simulink model "Motion_planner_Street_Drone"  (R2019b)
settings: Solver=FixedStepAuto  StartTime=0.0  StopTime=25  FixedStep=0.0075  MaxStep=1e-1  MinStep=1e-3  RelTol=1e-3  AbsTol=1e-4
InitFcn:
  | SD_init1
values from neighbouring files (symbols this model uses):
  cost = [2.71432892747 3.32441927977 3.79268757264 4.85642115368 6.12135035287 7.09825974303 9.57278659789 1.55754789407 1.51399555616 2.57723707661 3.8468529147 4.8336387623 ... (2430 elements, 1x2430)]    [matlab.mat]
  Front_brake = [0 2.2085352751 4.15209150797 6.12733711785 8.16604105928 9.79119154879 12.1808659635 14.1242630413 16.1155522836 18.1386900579 20.0839213981 22.1313006548 ... (68 elements, 34x2)]    [Front_brake.mat]
  N = size(X,1)    [curvature.m]
  obsx = [dx1 dx2 dx3 dx4]'    [dynamic_collison.m]    (also in dynamic_detection1.m = [x1 x2 x3 x4]')
  obsy = [dy1 dy2 dy3 dy4]'    [dynamic_collison.m]    (also in dynamic_detection1.m = [y1 y2 y3 y4]')
  x = obs_path(i,1)    [dynamic_collison.m]    (also in dynamic_detection1.m)
  X = [X]    [curvature.m]
  y = obs_path(i,2)    [dynamic_collison.m]    (also in dynamic_detection1.m)
undefined symbols (not defined in the file or in its folder): d, dfin, dini, Ki, Kp, L_0f, lookahead_time, lookahead_time_rev, Rear_brake, sigbuilder_block, steer_ratio, steer_sens, tfin, tini, TPS_0, xfin, Y, yfin, Z
libraries: sm_lib x290, nesl_utility x136, simulink x6, vrlib x2, powerlib_meascontrol x2
(part 12 of 14)

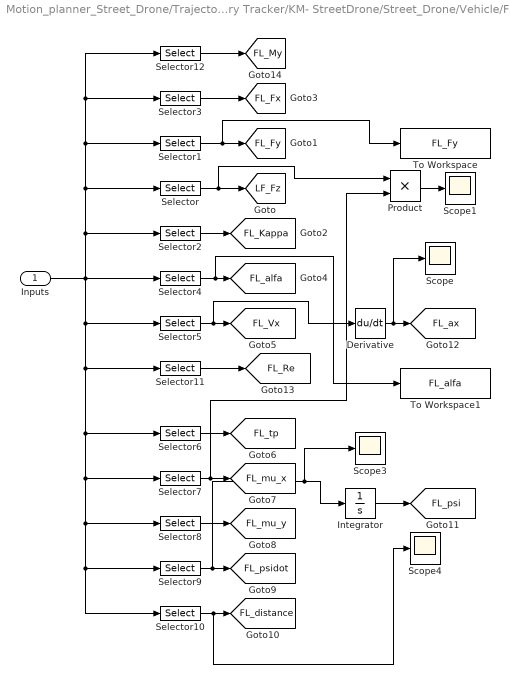
== system Motion_planner_Street_Drone/Trajectory Tracker/KM- StreetDrone/Street_Drone/Vehicle/FL_Wheel/For Validation ==
  Inputs : Inport
  Derivative : Derivative
  Integrator : Integrator
  Product : Product
  Scope{,1,3..4} (4 alike) : Scope
  Selector : Selector  InputPortWidth=40  IndexOptions=Index vector (dialog)  Indices=[3]  OutputSizes=1
  Selector1 : Selector  InputPortWidth=40  IndexOptions=Index vector (dialog)  Indices=[2]  OutputSizes=1
  Selector10 : Selector  InputPortWidth=40  IndexOptions=Index vector (dialog)  Indices=[28]  OutputSizes=1
  Selector11 : Selector  InputPortWidth=40  IndexOptions=Index vector (dialog)  Indices=[13]  OutputSizes=1
  Selector12 : Selector  InputPortWidth=40  IndexOptions=Index vector (dialog)  Indices=[5]  OutputSizes=1
  Selector2 : Selector  InputPortWidth=40  IndexOptions=Index vector (dialog)  Indices=[7]  OutputSizes=1
  Selector3 : Selector  InputPortWidth=40  IndexOptions=Index vector (dialog)  Indices=[1]  OutputSizes=1
  Selector4 : Selector  InputPortWidth=40  IndexOptions=Index vector (dialog)  Indices=[8]  OutputSizes=1
  Selector5 : Selector  InputPortWidth=40  IndexOptions=Index vector (dialog)  Indices=[11]  OutputSizes=1
  Selector6 : Selector  InputPortWidth=40  IndexOptions=Index vector (dialog)  Indices=[16]  OutputSizes=1
  Selector7 : Selector  InputPortWidth=40  IndexOptions=Index vector (dialog)  Indices=[17]  OutputSizes=1
  Selector8 : Selector  InputPortWidth=40  IndexOptions=Index vector (dialog)  Indices=[18]  OutputSizes=1
  Selector9 : Selector  InputPortWidth=40  IndexOptions=Index vector (dialog)  Indices=[24]  OutputSizes=1
  To Workspace : ToWorkspace  VariableName=FL_Fy  SampleTime=-1
  To Workspace1 : ToWorkspace  VariableName=FL_alfa  SampleTime=-1
  tag scope: FL_Fx=global, FL_Fy=global, FL_Kappa=global, FL_My=global, FL_Re=global, FL_Vx=global, FL_alfa=global, FL_ax=global, FL_distance=global, FL_mu_x=global, FL_mu_y=global, FL_psi=global, FL_psidot=global, FL_tp=global, LF_Fz=global
  wires:
  Selector12/1 -> [FL_My]
  Product/1 -> Scope1/1
  Derivative/1 -> [FL_ax], Scope/1
  Integrator/1 -> [FL_psi]
  Selector10/1 -> Scope4/1, [FL_distance]
  Inputs/1 -> Selector4/1, Selector2/1, Selector/1, Selector1/1, Selector3/1, Selector12/1, Selector5/1, Selector6/1, Selector7/1, Selector8/1, Selector9/1, Selector10/1, Selector11/1
  Selector9/1 -> [FL_psidot], Scope3/1, Integrator/1
  Selector8/1 -> [FL_mu_y]
  Selector7/1 -> [FL_mu_x], Product/2
  Selector6/1 -> [FL_tp]
  Selector5/1 -> [FL_Vx], Derivative/1
  Selector4/1 -> To Workspace1/1, [FL_alfa]
  Selector3/1 -> [FL_Fx]
  Selector2/1 -> [FL_Kappa]
  Selector1/1 -> To Workspace/1, [FL_Fy]
  Selector/1 -> [LF_Fz], Product/1
  Selector11/1 -> [FL_Re]

== system Motion_planner_Street_Drone/Trajectory Tracker/KM- StreetDrone/Street_Drone/Vehicle/FL_Wheel/Non-moving road ==
  omega2 : Constant  Value=zeros(18,1)
  road : Outport
  wires:
  omega2/1 -> road/1

== system Motion_planner_Street_Drone/Trajectory Tracker/KM- StreetDrone/Street_Drone/Vehicle/FL_Wheel/Scaling factors ==
  s_LKX : Constant  Value=LKX
  s_LKY : Constant  Value=LKY
  s_LKYC : Constant  Value=LKYC
  s_LKZC : Constant  Value=LKZC
  s_LMUX : Constant  Value=LMUX
  s_LMUY : Constant  Value=LMUY
  s_LTR : Constant  Value=LTR
  scaling_vector : Mux  Inputs=7
  scaling : Outport
  wires:
  s_LMUX/1 -> scaling_vector/1
  s_LKX/1 -> scaling_vector/2
  s_LMUY/1 -> scaling_vector/3
  s_LKY/1 -> scaling_vector/4
  s_LKYC/1 -> scaling_vector/5
  s_LTR/1 -> scaling_vector/6
  s_LKZC/1 -> scaling_vector/7
  scaling_vector/1 -> scaling/1

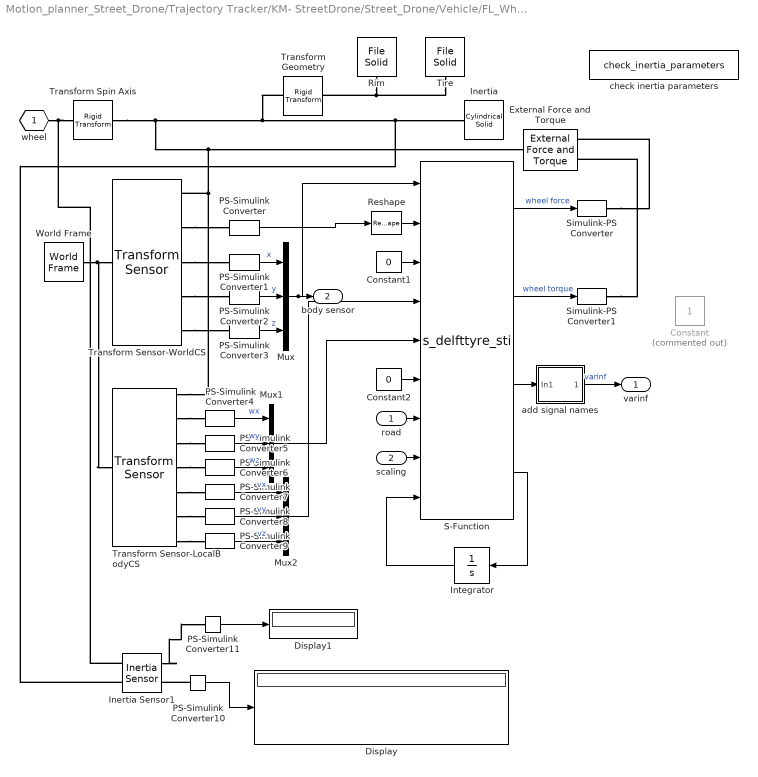
== system Motion_planner_Street_Drone/Trajectory Tracker/KM- StreetDrone/Street_Drone/Vehicle/FL_Wheel/SimMechanics2G Wheel + tyre ==
  road : Inport
  scaling : Inport  Port=2
  Constant : Constant  Commented=on
  Constant1 : Constant  Value=0
  Constant2 : Constant  Value=0
  Display : Display
  Display1 : Display
  External Force and Torque : sm_lib/Forces and Torques/External Force and Torque  ForceResolutionFrame=AttachedFrame  EnableForceX=off  EnableForceY=off  EnableForceZ=off  EnableForce=on  TorqueResolutionFrame=AttachedFrame  EnableTorqueX=off  EnableTorqueY=off  EnableTorqueZ=off  EnableTorque=on
  Inertia : sm_lib/Body Elements/Cylindrical Solid  GraphicAmbientColor=[0.15 0.15 0.15 1.0]  BasedOnType=Density  CenterOfMass=[0 0 0]  CenterOfMassUnits=m  GraphicDiffuseColor=[0.2 0.8 1.0]  CylinderLength=0.001  CylinderLengthUnits=m  CylinderRadius=0.001  CylinderRadiusUnits=m  Density=1000  DensityUnits=kg/(m^3)  DoExposeReferenceFrame=on  GraphicEmissiveColor=[0.0 0.0 0.0 1.0]  ExportEntireGeometry=off  SerializedFrames=<Frames/>  MarkerShape=Sphere  MarkerSize=10  GraphicType=FromGeometry  InertiaType=Custom  Mass=mass  MassUnits=kg  MomentsOfInertia=[Imat(1,1) Imat(2,2) Imat(3,3)]  MomentsOfInertiaUnits=kg*m^2  GraphicOpacity=1.0  ProductsOfInertia=[0 0 0]  ProductsOfInertiaUnits=kg*m^2  GraphicShininess=75  GraphicSpecularColor=[0.5 0.5 0.5 1.0]  GraphicVisPropType=SimpleVisualProperties
  Inertia Sensor1 : sm_lib/Body Elements/Inertia Sensor  SensorExtent=BodyGroup  SpanWeldJoints=off  ExcludeGroundedBodies=off  MeasurementFrame=Custom  SenseMass=on  SenseCenterOfMass=off  SenseInertiaMatrix=on  SenseCenteredInertiaMatrix=off  SensePrincipalInertiaMatrix=off  SenseRotationMatrix=off  GraphicType=PrincipalInertiaFrame  PrincipalInertiaFrameSize=20  GraphicVisPropType=SimpleVisualProperties  GraphicDiffuseColor=[0.5 0.5 0.5]  GraphicSpecularColor=[0.5 0.5 0.5 1.0]  GraphicAmbientColor=[0.15 0.15 0.15 1.0]  GraphicEmissiveColor=[0.0 0.0 0.0 1.0]  GraphicShininess=75  GraphicOpacity=1.0
      settings: SourceProductBaseCode=MS
  Integrator : Integrator  InitialCondition=zeros(1,40)
  Mux : Mux  Inputs=3
  Mux1 : Mux  Inputs=3
  Mux2 : Mux  Inputs=3
  PS-Simulink Converter{,1..9} (10 alike) : nesl_utility/PS-Simulink Converter  PhysicalDomain=network_engine_domain  SubClassName=ps_output  LeftPortType=input  RightPortType=output  PseudoPeriodic=off  Frequencies=[]  Unit=1  AffineConversion=off
  PS-Simulink Converter10 : nesl_utility/PS-Simulink Converter  PhysicalDomain=network_engine_domain  SubClassName=ps_output  LeftPortType=input  RightPortType=output  PseudoPeriodic=off  Frequencies=[]  Unit=inherit  AffineConversion=off
  PS-Simulink Converter11 : nesl_utility/PS-Simulink Converter  PhysicalDomain=network_engine_domain  SubClassName=ps_output  LeftPortType=input  RightPortType=output  PseudoPeriodic=off  Frequencies=[]  Unit=inherit  AffineConversion=off
  Reshape : Reshape
  Rim : sm_lib/Body Elements/File Solid  ExtGeomFileName=D:\Project\PATH PLANNER STREET DRONE - 618341\CAD geometry\Rim_Front.stl  UnitType=Custom  ExtGeomFileUnits=mm  StepReaderType=HEX  ExportEntireGeometry=off  InertiaType=Custom  Mass=0  MassUnits=kg  CenterOfMass=[0 0 0]  CenterOfMassUnits=m  MomentsOfInertia=[0 0 0]  MomentsOfInertiaUnits=kg*m^2  ProductsOfInertia=[0 0 0]  ProductsOfInertiaUnits=kg*m^2  BasedOnType=Density  Density=1000  DensityUnits=kg/(m^3)  DoExposeReferenceFrame=on  SerializedFrames=<Frames/>  GraphicType=FromGeometry  MarkerShape=Sphere  MarkerSize=10  MarkerSizeUnits=m  GraphicVisPropType=SimpleVisualProperties  GraphicDiffuseColor=[0.8 0.8 0.8]  GraphicSpecularColor=[0.5 0.5 0.5 1.0]  GraphicAmbientColor=[0.15 0.15 0.15 1.0]  GraphicEmissiveColor=[0.0 0.0 0.0 1.0]  GraphicShininess=75  GraphicOpacity=1.0
  S-Function : S-Function  FunctionName=s_delfttyre_sti  Parameters=iswtch idtyre idroad tpfname_dummy rdfname typarr  SFunctionDeploymentMode=off  EnableBusSupport=off
  Simulink-PS Converter : nesl_utility/Simulink-PS Converter  PhysicalDomain=network_engine_domain  SubClassName=ps_input  LeftPortType=input  RightPortType=output  PseudoPeriodic=off  Frequencies=[]  NoiseDistribution=none  NoiseParameters=[]  Unit=1  AffineConversion=off  FilteringAndDerivatives=zero  SimscapeFilterOrder=1  InputFilterTimeConstant=0.001  UdotUserProvided=1
  Simulink-PS Converter1 : nesl_utility/Simulink-PS Converter  PhysicalDomain=network_engine_domain  SubClassName=ps_input  LeftPortType=input  RightPortType=output  PseudoPeriodic=off  Frequencies=[]  NoiseDistribution=none  NoiseParameters=[]  Unit=1  AffineConversion=off  FilteringAndDerivatives=zero  SimscapeFilterOrder=1  InputFilterTimeConstant=0.001  UdotUserProvided=1
  Tire : sm_lib/Body Elements/File Solid  ExtGeomFileName=D:\Project\PATH PLANNER STREET DRONE - 618341\CAD geometry\Tire_Front.stl  UnitType=Custom  ExtGeomFileUnits=mm  StepReaderType=HEX  ExportEntireGeometry=off  InertiaType=Custom  Mass=0  MassUnits=kg  CenterOfMass=[0 0 0]  CenterOfMassUnits=m  MomentsOfInertia=[0 0 0]  MomentsOfInertiaUnits=kg*m^2  ProductsOfInertia=[0 0 0]  ProductsOfInertiaUnits=kg*m^2  BasedOnType=Density  Density=1000  DensityUnits=kg/(m^3)  DoExposeReferenceFrame=on  SerializedFrames=<Frames/>  GraphicType=FromGeometry  MarkerShape=Sphere  MarkerSize=10  MarkerSizeUnits=m  GraphicVisPropType=SimpleVisualProperties  GraphicDiffuseColor=[0.5 0.5 0.5]  GraphicSpecularColor=[0.5 0.5 0.5 1.0]  GraphicAmbientColor=[0.15 0.15 0.15 1.0]  GraphicEmissiveColor=[0.0 0.0 0.0 1.0]  GraphicShininess=75  GraphicOpacity=1.0
  Transform Geometry : sm_lib/Frames and Transforms/Rigid Transform  TranslationMethod=StandardAxis  TranslationStandardOffset=(1-2*fliplr)*0.125  TranslationLengthUnit=m  TranslationStandardAxis=+Y  TranslationCartesianOffset=[0 0 0]  TranslationROffset=0  TranslationROffsetUnits=m  TranslationZOffset=0  TranslationZOffsetUnits=m  TranslationThetaOffset=0  TranslationThetaOffsetUnits=deg  RotationMethod=StandardAxis  RotationAngleUnits=deg  RotationStandardAxis=+X  RotationAngle=fliplr*180-90  RotationArbitraryAxis=[0 0 1]  FollAlignAxisA=+X  BaseAlignAxisA=+Y  FollAlignAxisB=+Y  BaseAlignAxisB=+Z  RotationSequenceAxes=FollowerAxes  RotationSequence=XYX  RotationSequenceAngles=[0 0 0]  RotationSequenceAnglesUnits=deg  RotationMatrix=[1 0 0; 0 1 0; 0 0 1]
  Transform Sensor-LocalBodyCS : sm_lib/Frames and Transforms/Transform Sensor  MeasurementFrame=NonRotatingFollower  SenseAngle=off  SenseAxis=off  SenseAngle1=off  SenseAngle2=off  SenseAngle3=off  SenseQ=off  SenseR=off  SenseOmegaX=on  SenseOmegaY=on  SenseOmegaZ=on  SenseOmega1=off  SenseOmega2=off  SenseOmega3=off  SenseQDot=off  SenseRDot=off  SenseAlphaX=off  SenseAlphaY=off  SenseAlphaZ=off  SenseAlpha1=off  SenseAlpha2=off  SenseAlpha3=off  SenseQDDot=off  SenseRDDot=off  SenseX=off  SenseY=off  SenseZ=off  SenseRad=off  SenseAzim=off  SenseDist=off  SenseInc=off  SenseXDot=on  SenseYDot=on  SenseZDot=on  SenseRadDot=off  SenseAzimDot=off  SenseDistDot=off  SenseIncDot=off  SenseXDDot=off  SenseYDDot=off  SenseZDDot=off  SenseRadDDot=off  SenseAzimDDot=off  SenseDistDDot=off  SenseIncDDot=off
  Transform Sensor-WorldCS : sm_lib/Frames and Transforms/Transform Sensor  MeasurementFrame=World  SenseAngle=off  SenseAxis=off  SenseAngle1=off  SenseAngle2=off  SenseAngle3=off  SenseQ=off  SenseR=on  SenseOmegaX=off  SenseOmegaY=off  SenseOmegaZ=off  SenseOmega1=off  SenseOmega2=off  SenseOmega3=off  SenseQDot=off  SenseRDot=off  SenseAlphaX=off  SenseAlphaY=off  SenseAlphaZ=off  SenseAlpha1=off  SenseAlpha2=off  SenseAlpha3=off  SenseQDDot=off  SenseRDDot=off  SenseX=on  SenseY=on  SenseZ=on  SenseRad=off  SenseAzim=off  SenseDist=off  SenseInc=off  SenseXDot=off  SenseYDot=off  SenseZDot=off  SenseRadDot=off  SenseAzimDot=off  SenseDistDot=off  SenseIncDot=off  SenseXDDot=off  SenseYDDot=off  SenseZDDot=off  SenseRadDDot=off  SenseAzimDDot=off  SenseDistDDot=off  SenseIncDDot=off
  Transform Spin Axis : sm_lib/Frames and Transforms/Rigid Transform  TranslationMethod=None  TranslationStandardOffset=0  TranslationLengthUnit=m  TranslationStandardAxis=+Z  TranslationCartesianOffset=[0 0 0]  TranslationROffset=0  TranslationROffsetUnits=m  TranslationZOffset=0  TranslationZOffsetUnits=m  TranslationThetaOffset=0  TranslationThetaOffsetUnits=deg  RotationMethod=StandardAxis  RotationAngleUnits=deg  RotationStandardAxis=-X  RotationAngle=90  RotationArbitraryAxis=[0 0 1]  FollAlignAxisA=+X  BaseAlignAxisA=+Y  FollAlignAxisB=+Y  BaseAlignAxisB=+Z  RotationSequenceAxes=FollowerAxes  RotationSequence=XYX  RotationSequenceAngles=[0 0 0]  RotationSequenceAnglesUnits=deg  RotationMatrix=[1 0 0; 0 1 0; 0 0 1]
  World Frame : sm_lib/Frames and Transforms/World Frame
  add signal names : Subsystem
  check inertia parameters : M-S-Function  Priority=1  FunctionName=check_inertia_parameters  Parameters=tpfname1, rdfname1, typarr1  mask{tpfname1=tpfname_dummy, rdfname1=rdfname, typarr1=typarr}
      mask prompts: tpfname1 "Tyre Property File"; rdfname1 "Road Data File"; typarr1 "typarr"
      mask help: Checks Inertia parameters as calculated in mask
  wheel : PMIOPort  Side=Left
  varinf : Outport
  body sensor : Outport  Port=2
  wires:
  PS-Simulink Converter11/1 -> Display1/1
  PS-Simulink Converter10/1 -> Display/1
  Constant2/1 -> S-Function/6
  Mux2/1 -> S-Function/4
  Mux1/1 -> S-Function/5
  PS-Simulink Converter/1 -> Reshape/1
  S-Function/4 -> Integrator/1
  S-Function/3 -> add signal names/1(In1)
  add signal names/1(Out1) -> varinf/1  "varinf"
  road/1 -> S-Function/7
  scaling/1 -> S-Function/8
  Integrator/1 -> S-Function/9
  Constant1/1 -> S-Function/3
  PS-Simulink Converter1/1 -> Mux/1  "x"
  PS-Simulink Converter2/1 -> Mux/2  "y"
  PS-Simulink Converter3/1 -> Mux/3  "z"
  PS-Simulink Converter4/1 -> Mux1/1  "wx"
  PS-Simulink Converter5/1 -> Mux1/2  "wy"
  PS-Simulink Converter6/1 -> Mux1/3  "wz"
  PS-Simulink Converter7/1 -> Mux2/1  "vx"
  PS-Simulink Converter8/1 -> Mux2/2  "vy"
  PS-Simulink Converter9/1 -> Mux2/3  "vz"
  Mux/1 -> body sensor/1, S-Function/1
  S-Function/2 -> Simulink-PS Converter1/1  "wheel torque"
  S-Function/1 -> Simulink-PS Converter/1  "wheel force"
  Reshape/1 -> S-Function/2
  connections:
  Inertia Sensor1/RConn1 -- PS-Simulink Converter11/LConn1
  PS-Simulink Converter10/LConn1 -- Inertia Sensor1/RConn2
  Inertia Sensor1/LConn1 -- wheel/RConn1 -- Transform Spin Axis/RConn1
  Simulink-PS Converter1/RConn1 -- External Force and Torque/LConn2
  Simulink-PS Converter/RConn1 -- External Force and Torque/LConn1
  Transform Sensor-WorldCS/RConn2 -- PS-Simulink Converter/LConn1
  Transform Sensor-WorldCS/RConn3 -- PS-Simulink Converter1/LConn1
  Transform Sensor-WorldCS/RConn4 -- PS-Simulink Converter2/LConn1
  Transform Sensor-WorldCS/RConn5 -- PS-Simulink Converter3/LConn1
  Transform Sensor-LocalBodyCS/RConn2 -- PS-Simulink Converter4/LConn1
  Transform Sensor-LocalBodyCS/RConn3 -- PS-Simulink Converter5/LConn1
  Transform Sensor-LocalBodyCS/RConn4 -- PS-Simulink Converter6/LConn1
  Transform Sensor-LocalBodyCS/RConn5 -- PS-Simulink Converter7/LConn1
  Transform Sensor-LocalBodyCS/RConn6 -- PS-Simulink Converter8/LConn1
  Transform Sensor-LocalBodyCS/RConn7 -- PS-Simulink Converter9/LConn1
  Tire/RConn1 -- Rim/RConn1 -- Transform Geometry/RConn1
  Inertia Sensor1/LConn2 -- Transform Geometry/LConn1 -- External Force and Torque/RConn1 -- Transform Sensor-LocalBodyCS/RConn1 -- Transform Sensor-WorldCS/RConn1 -- Transform Spin Axis/LConn1 -- Inertia/RConn1
  Transform Sensor-LocalBodyCS/LConn1 -- World Frame/RConn1 -- Transform Sensor-WorldCS/LConn1

== system Motion_planner_Street_Drone/Trajectory Tracker/KM- StreetDrone/Street_Drone/Vehicle/FR_Suspension/steering_angle_measurement ==
  Integrator1 : Integrator
  PS-Simulink Converter3 : nesl_utility/PS-Simulink Converter  PhysicalDomain=network_engine_domain  SubClassName=ps_output  LeftPortType=input  RightPortType=output  PseudoPeriodic=off  Frequencies=[]  Unit=inherit  AffineConversion=off
  PS-Simulink Converter4 : nesl_utility/PS-Simulink Converter  PhysicalDomain=network_engine_domain  SubClassName=ps_output  LeftPortType=input  RightPortType=output  PseudoPeriodic=off  Frequencies=[]  Unit=inherit  AffineConversion=off
  Scope2 : Scope  NumInputPorts=2
  Transform Sensor2 : sm_lib/Frames and Transforms/Transform Sensor  MeasurementFrame=Base  SenseAngle=off  SenseAxis=off  SenseAngle1=off  SenseAngle2=off  SenseAngle3=off  SenseQ=off  SenseR=off  SenseOmegaX=off  SenseOmegaY=on  SenseOmegaZ=on  SenseOmega1=off  SenseOmega2=off  SenseOmega3=off  SenseQDot=off  SenseRDot=off  SenseAlphaX=off  SenseAlphaY=off  SenseAlphaZ=off  SenseAlpha1=off  SenseAlpha2=off  SenseAlpha3=off  SenseQDDot=off  SenseRDDot=off  SenseX=off  SenseY=off  SenseZ=off  SenseRad=off  SenseAzim=off  SenseDist=off  SenseInc=off  SenseXDot=off  SenseYDot=off  SenseZDot=off  SenseRadDot=off  SenseAzimDot=off  SenseDistDot=off  SenseIncDot=off  SenseXDDot=off  SenseYDDot=off  SenseZDDot=off  SenseRadDDot=off  SenseAzimDDot=off  SenseDistDDot=off  SenseIncDDot=off
  vehicle : PMIOPort  Side=Left
  suspension_z-axis : PMIOPort  Port=2  Side=Right
  tag scope: Del_R=global
  wires:
  PS-Simulink Converter3/1 -> Integrator1/1
  PS-Simulink Converter4/1 -> Scope2/1
  Integrator1/1 -> Scope2/2, [Del_R]
  connections:
  PS-Simulink Converter4/LConn1 -- Transform Sensor2/RConn2
  suspension_z-axis/RConn1 -- Transform Sensor2/RConn1
  Transform Sensor2/LConn1 -- vehicle/RConn1
  PS-Simulink Converter3/LConn1 -- Transform Sensor2/RConn3

== system Motion_planner_Street_Drone/Trajectory Tracker/KM- StreetDrone/Street_Drone/Vehicle/FR_Wheel/For Validation ==
  Inputs : Inport
  Derivative : Derivative
  Integrator : Integrator
  Scope : Scope
  Selector : Selector  InputPortWidth=40  IndexOptions=Index vector (dialog)  Indices=[3]  OutputSizes=1
  Selector1 : Selector  InputPortWidth=40  IndexOptions=Index vector (dialog)  Indices=[2]  OutputSizes=1
  Selector10 : Selector  InputPortWidth=40  IndexOptions=Index vector (dialog)  Indices=[28]  OutputSizes=1
  Selector11 : Selector  InputPortWidth=40  IndexOptions=Index vector (dialog)  Indices=[13]  OutputSizes=1
  Selector12 : Selector  InputPortWidth=40  IndexOptions=Index vector (dialog)  Indices=[5]  OutputSizes=1
  Selector2 : Selector  InputPortWidth=40  IndexOptions=Index vector (dialog)  Indices=[7]  OutputSizes=1
  Selector3 : Selector  InputPortWidth=40  IndexOptions=Index vector (dialog)  Indices=[1]  OutputSizes=1
  Selector4 : Selector  InputPortWidth=40  IndexOptions=Index vector (dialog)  Indices=[8]  OutputSizes=1
  Selector5 : Selector  InputPortWidth=40  IndexOptions=Index vector (dialog)  Indices=[11]  OutputSizes=1
  Selector6 : Selector  InputPortWidth=40  IndexOptions=Index vector (dialog)  Indices=[16]  OutputSizes=1
  Selector7 : Selector  InputPortWidth=40  IndexOptions=Index vector (dialog)  Indices=[17]  OutputSizes=1
  Selector8 : Selector  InputPortWidth=40  IndexOptions=Index vector (dialog)  Indices=[18]  OutputSizes=1
  Selector9 : Selector  InputPortWidth=40  IndexOptions=Index vector (dialog)  Indices=[24]  OutputSizes=1
  tag scope: FR_Fx=global, FR_Fy=global, FR_Kappa=global, FR_My=global, FR_Re=global, FR_Vx=global, FR_alfa=global, FR_ax=global, FR_distance=global, FR_mu_x=global, FR_mu_y=global, FR_psi=global, FR_psidot=global, FR_tp=global, RF_Fz=global
  wires:
  Selector12/1 -> [FR_My]
  Derivative/1 -> [FR_ax]
  Integrator/1 -> [FR_psi]
  Selector10/1 -> [FR_distance]
  Inputs/1 -> Selector4/1, Selector2/1, Selector/1, Selector1/1, Selector3/1, Selector12/1, Selector5/1, Selector11/1, Selector6/1, Selector7/1, Selector8/1, Selector9/1, Selector10/1
  Selector9/1 -> [FR_psidot], Scope/1, Integrator/1
  Selector8/1 -> [FR_mu_y]
  Selector7/1 -> [FR_mu_x]
  Selector6/1 -> [FR_tp]
  Selector5/1 -> [FR_Vx], Derivative/1
  Selector4/1 -> [FR_alfa]
  Selector3/1 -> [FR_Fx]
  Selector2/1 -> [FR_Kappa]
  Selector1/1 -> [FR_Fy]
  Selector/1 -> [RF_Fz]
  Selector11/1 -> [FR_Re]

== system Motion_planner_Street_Drone/Trajectory Tracker/KM- StreetDrone/Street_Drone/Vehicle/FR_Wheel/Non-moving road ==
  omega2 : Constant  Value=zeros(18,1)
  road : Outport
  wires:
  omega2/1 -> road/1

== system Motion_planner_Street_Drone/Trajectory Tracker/KM- StreetDrone/Street_Drone/Vehicle/FR_Wheel/Scaling factors ==
  s_LKX : Constant  Value=LKX
  s_LKY : Constant  Value=LKY
  s_LKYC : Constant  Value=LKYC
  s_LKZC : Constant  Value=LKZC
  s_LMUX : Constant  Value=LMUX
  s_LMUY : Constant  Value=LMUY
  s_LTR : Constant  Value=LTR
  scaling_vector : Mux  Inputs=7
  scaling : Outport
  wires:
  scaling_vector/1 -> scaling/1
  s_LKZC/1 -> scaling_vector/7
  s_LTR/1 -> scaling_vector/6
  s_LKYC/1 -> scaling_vector/5
  s_LKY/1 -> scaling_vector/4
  s_LMUY/1 -> scaling_vector/3
  s_LKX/1 -> scaling_vector/2
  s_LMUX/1 -> scaling_vector/1

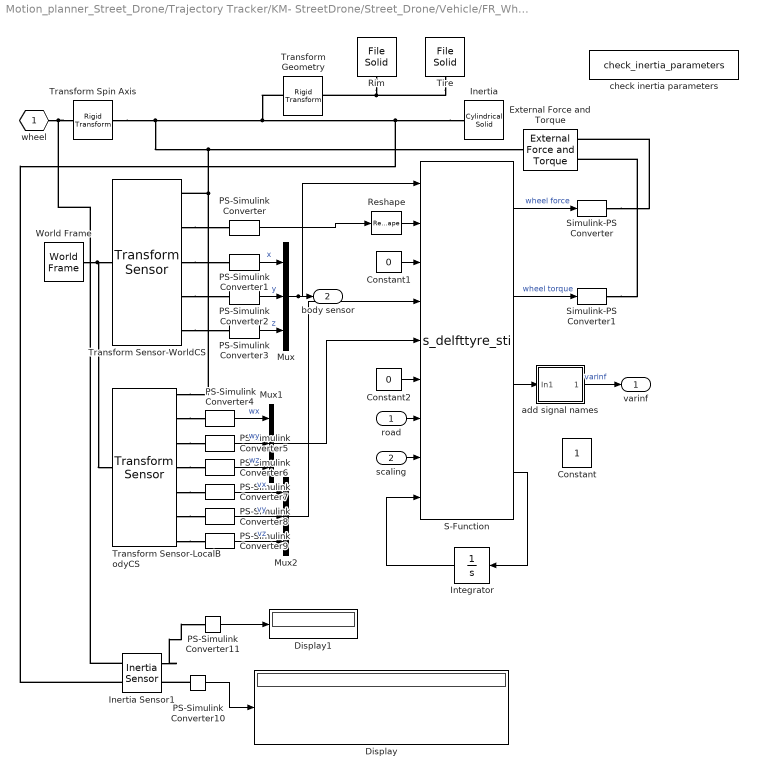
== system Motion_planner_Street_Drone/Trajectory Tracker/KM- StreetDrone/Street_Drone/Vehicle/FR_Wheel/SimMechanics2G Wheel + tyre ==
  road : Inport
  scaling : Inport  Port=2
  Constant : Constant
  Constant1 : Constant  Value=0
  Constant2 : Constant  Value=0
  Display : Display
  Display1 : Display
  External Force and Torque : sm_lib/Forces and Torques/External Force and Torque  ForceResolutionFrame=AttachedFrame  EnableForceX=off  EnableForceY=off  EnableForceZ=off  EnableForce=on  TorqueResolutionFrame=AttachedFrame  EnableTorqueX=off  EnableTorqueY=off  EnableTorqueZ=off  EnableTorque=on
  Inertia : sm_lib/Body Elements/Cylindrical Solid  GraphicAmbientColor=[0.15 0.15 0.15 1.0]  BasedOnType=Density  CenterOfMass=[0 0 0]  CenterOfMassUnits=m  GraphicDiffuseColor=[0.2 0.8 1.0]  CylinderLength=0.001  CylinderLengthUnits=m  CylinderRadius=0.001  CylinderRadiusUnits=m  Density=1000  DensityUnits=kg/(m^3)  DoExposeReferenceFrame=on  GraphicEmissiveColor=[0.0 0.0 0.0 1.0]  ExportEntireGeometry=off  SerializedFrames=<Frames/>  MarkerShape=Sphere  MarkerSize=10  GraphicType=FromGeometry  InertiaType=Custom  Mass=mass  MassUnits=kg  MomentsOfInertia=[Imat(1,1) Imat(2,2) Imat(3,3)]  MomentsOfInertiaUnits=kg*m^2  GraphicOpacity=1.0  ProductsOfInertia=[0 0 0]  ProductsOfInertiaUnits=kg*m^2  GraphicShininess=75  GraphicSpecularColor=[0.5 0.5 0.5 1.0]  GraphicVisPropType=SimpleVisualProperties
  Inertia Sensor1 : sm_lib/Body Elements/Inertia Sensor  SensorExtent=BodyGroup  SpanWeldJoints=off  ExcludeGroundedBodies=off  MeasurementFrame=Custom  SenseMass=on  SenseCenterOfMass=off  SenseInertiaMatrix=on  SenseCenteredInertiaMatrix=off  SensePrincipalInertiaMatrix=off  SenseRotationMatrix=off  GraphicType=PrincipalInertiaFrame  PrincipalInertiaFrameSize=20  GraphicVisPropType=SimpleVisualProperties  GraphicDiffuseColor=[0.5 0.5 0.5]  GraphicSpecularColor=[0.5 0.5 0.5 1.0]  GraphicAmbientColor=[0.15 0.15 0.15 1.0]  GraphicEmissiveColor=[0.0 0.0 0.0 1.0]  GraphicShininess=75  GraphicOpacity=1.0
      settings: SourceProductBaseCode=MS
  Integrator : Integrator  InitialCondition=zeros(1,40)
  Mux : Mux  Inputs=3
  Mux1 : Mux  Inputs=3
  Mux2 : Mux  Inputs=3
  PS-Simulink Converter{,1..9} (10 alike) : nesl_utility/PS-Simulink Converter  PhysicalDomain=network_engine_domain  SubClassName=ps_output  LeftPortType=input  RightPortType=output  PseudoPeriodic=off  Frequencies=[]  Unit=1  AffineConversion=off
  PS-Simulink Converter10 : nesl_utility/PS-Simulink Converter  PhysicalDomain=network_engine_domain  SubClassName=ps_output  LeftPortType=input  RightPortType=output  PseudoPeriodic=off  Frequencies=[]  Unit=inherit  AffineConversion=off
  PS-Simulink Converter11 : nesl_utility/PS-Simulink Converter  PhysicalDomain=network_engine_domain  SubClassName=ps_output  LeftPortType=input  RightPortType=output  PseudoPeriodic=off  Frequencies=[]  Unit=inherit  AffineConversion=off
  Reshape : Reshape
  Rim : sm_lib/Body Elements/File Solid  ExtGeomFileName=D:\Project\PATH PLANNER STREET DRONE - 618341\CAD geometry\Rim_Front.stl  UnitType=Custom  ExtGeomFileUnits=mm  StepReaderType=HEX  ExportEntireGeometry=off  InertiaType=Custom  Mass=0  MassUnits=kg  CenterOfMass=[0 0 0]  CenterOfMassUnits=m  MomentsOfInertia=[0 0 0]  MomentsOfInertiaUnits=kg*m^2  ProductsOfInertia=[0 0 0]  ProductsOfInertiaUnits=kg*m^2  BasedOnType=Density  Density=1000  DensityUnits=kg/(m^3)  DoExposeReferenceFrame=on  SerializedFrames=<Frames/>  GraphicType=FromGeometry  MarkerShape=Sphere  MarkerSize=10  MarkerSizeUnits=m  GraphicVisPropType=SimpleVisualProperties  GraphicDiffuseColor=[0.8 0.8 0.8]  GraphicSpecularColor=[0.5 0.5 0.5 1.0]  GraphicAmbientColor=[0.15 0.15 0.15 1.0]  GraphicEmissiveColor=[0.0 0.0 0.0 1.0]  GraphicShininess=75  GraphicOpacity=1.0
  S-Function : S-Function  FunctionName=s_delfttyre_sti  Parameters=iswtch idtyre idroad tpfname_dummy rdfname typarr  SFunctionDeploymentMode=off  EnableBusSupport=off
  Simulink-PS Converter : nesl_utility/Simulink-PS Converter  PhysicalDomain=network_engine_domain  SubClassName=ps_input  LeftPortType=input  RightPortType=output  PseudoPeriodic=off  Frequencies=[]  NoiseDistribution=none  NoiseParameters=[]  Unit=1  AffineConversion=off  FilteringAndDerivatives=zero  SimscapeFilterOrder=1  InputFilterTimeConstant=0.001  UdotUserProvided=1
  Simulink-PS Converter1 : nesl_utility/Simulink-PS Converter  PhysicalDomain=network_engine_domain  SubClassName=ps_input  LeftPortType=input  RightPortType=output  PseudoPeriodic=off  Frequencies=[]  NoiseDistribution=none  NoiseParameters=[]  Unit=1  AffineConversion=off  FilteringAndDerivatives=zero  SimscapeFilterOrder=1  InputFilterTimeConstant=0.001  UdotUserProvided=1
  Tire : sm_lib/Body Elements/File Solid  ExtGeomFileName=D:\Project\PATH PLANNER STREET DRONE - 618341\CAD geometry\Tire_Front.stl  UnitType=Custom  ExtGeomFileUnits=mm  StepReaderType=HEX  ExportEntireGeometry=off  InertiaType=Custom  Mass=0  MassUnits=kg  CenterOfMass=[0 0 0]  CenterOfMassUnits=m  MomentsOfInertia=[0 0 0]  MomentsOfInertiaUnits=kg*m^2  ProductsOfInertia=[0 0 0]  ProductsOfInertiaUnits=kg*m^2  BasedOnType=Density  Density=1000  DensityUnits=kg/(m^3)  DoExposeReferenceFrame=on  SerializedFrames=<Frames/>  GraphicType=FromGeometry  MarkerShape=Sphere  MarkerSize=10  MarkerSizeUnits=m  GraphicVisPropType=SimpleVisualProperties  GraphicDiffuseColor=[0.5 0.5 0.5]  GraphicSpecularColor=[0.5 0.5 0.5 1.0]  GraphicAmbientColor=[0.15 0.15 0.15 1.0]  GraphicEmissiveColor=[0.0 0.0 0.0 1.0]  GraphicShininess=75  GraphicOpacity=1.0
  Transform Geometry : sm_lib/Frames and Transforms/Rigid Transform  TranslationMethod=StandardAxis  TranslationStandardOffset=(1-2*fliplr)*0.125  TranslationLengthUnit=m  TranslationStandardAxis=+Y  TranslationCartesianOffset=[0 0 0]  TranslationROffset=0  TranslationROffsetUnits=m  TranslationZOffset=0  TranslationZOffsetUnits=m  TranslationThetaOffset=0  TranslationThetaOffsetUnits=deg  RotationMethod=StandardAxis  RotationAngleUnits=deg  RotationStandardAxis=+X  RotationAngle=fliplr*180-90  RotationArbitraryAxis=[0 0 1]  FollAlignAxisA=+X  BaseAlignAxisA=+Y  FollAlignAxisB=+Y  BaseAlignAxisB=+Z  RotationSequenceAxes=FollowerAxes  RotationSequence=XYX  RotationSequenceAngles=[0 0 0]  RotationSequenceAnglesUnits=deg  RotationMatrix=[1 0 0; 0 1 0; 0 0 1]
  Transform Sensor-LocalBodyCS : sm_lib/Frames and Transforms/Transform Sensor  MeasurementFrame=NonRotatingFollower  SenseAngle=off  SenseAxis=off  SenseAngle1=off  SenseAngle2=off  SenseAngle3=off  SenseQ=off  SenseR=off  SenseOmegaX=on  SenseOmegaY=on  SenseOmegaZ=on  SenseOmega1=off  SenseOmega2=off  SenseOmega3=off  SenseQDot=off  SenseRDot=off  SenseAlphaX=off  SenseAlphaY=off  SenseAlphaZ=off  SenseAlpha1=off  SenseAlpha2=off  SenseAlpha3=off  SenseQDDot=off  SenseRDDot=off  SenseX=off  SenseY=off  SenseZ=off  SenseRad=off  SenseAzim=off  SenseDist=off  SenseInc=off  SenseXDot=on  SenseYDot=on  SenseZDot=on  SenseRadDot=off  SenseAzimDot=off  SenseDistDot=off  SenseIncDot=off  SenseXDDot=off  SenseYDDot=off  SenseZDDot=off  SenseRadDDot=off  SenseAzimDDot=off  SenseDistDDot=off  SenseIncDDot=off
  Transform Sensor-WorldCS : sm_lib/Frames and Transforms/Transform Sensor  MeasurementFrame=World  SenseAngle=off  SenseAxis=off  SenseAngle1=off  SenseAngle2=off  SenseAngle3=off  SenseQ=off  SenseR=on  SenseOmegaX=off  SenseOmegaY=off  SenseOmegaZ=off  SenseOmega1=off  SenseOmega2=off  SenseOmega3=off  SenseQDot=off  SenseRDot=off  SenseAlphaX=off  SenseAlphaY=off  SenseAlphaZ=off  SenseAlpha1=off  SenseAlpha2=off  SenseAlpha3=off  SenseQDDot=off  SenseRDDot=off  SenseX=on  SenseY=on  SenseZ=on  SenseRad=off  SenseAzim=off  SenseDist=off  SenseInc=off  SenseXDot=off  SenseYDot=off  SenseZDot=off  SenseRadDot=off  SenseAzimDot=off  SenseDistDot=off  SenseIncDot=off  SenseXDDot=off  SenseYDDot=off  SenseZDDot=off  SenseRadDDot=off  SenseAzimDDot=off  SenseDistDDot=off  SenseIncDDot=off
  Transform Spin Axis : sm_lib/Frames and Transforms/Rigid Transform  TranslationMethod=None  TranslationStandardOffset=0  TranslationLengthUnit=m  TranslationStandardAxis=+Z  TranslationCartesianOffset=[0 0 0]  TranslationROffset=0  TranslationROffsetUnits=m  TranslationZOffset=0  TranslationZOffsetUnits=m  TranslationThetaOffset=0  TranslationThetaOffsetUnits=deg  RotationMethod=StandardAxis  RotationAngleUnits=deg  RotationStandardAxis=-X  RotationAngle=90  RotationArbitraryAxis=[0 0 1]  FollAlignAxisA=+X  BaseAlignAxisA=+Y  FollAlignAxisB=+Y  BaseAlignAxisB=+Z  RotationSequenceAxes=FollowerAxes  RotationSequence=XYX  RotationSequenceAngles=[0 0 0]  RotationSequenceAnglesUnits=deg  RotationMatrix=[1 0 0; 0 1 0; 0 0 1]
  World Frame : sm_lib/Frames and Transforms/World Frame
  add signal names : Subsystem
  check inertia parameters : M-S-Function  Priority=1  FunctionName=check_inertia_parameters  Parameters=tpfname1, rdfname1, typarr1  mask{tpfname1=tpfname_dummy, rdfname1=rdfname, typarr1=typarr}
      mask prompts: tpfname1 "Tyre Property File"; rdfname1 "Road Data File"; typarr1 "typarr"
      mask help: Checks Inertia parameters as calculated in mask
  wheel : PMIOPort  Side=Left
  varinf : Outport
  body sensor : Outport  Port=2
  wires:
  Reshape/1 -> S-Function/2
  S-Function/1 -> Simulink-PS Converter/1  "wheel force"
  S-Function/2 -> Simulink-PS Converter1/1  "wheel torque"
  Mux/1 -> S-Function/1, body sensor/1
  PS-Simulink Converter9/1 -> Mux2/3  "vz"
  PS-Simulink Converter8/1 -> Mux2/2  "vy"
  PS-Simulink Converter7/1 -> Mux2/1  "vx"
  PS-Simulink Converter6/1 -> Mux1/3  "wz"
  PS-Simulink Converter5/1 -> Mux1/2  "wy"
  PS-Simulink Converter4/1 -> Mux1/1  "wx"
  PS-Simulink Converter3/1 -> Mux/3  "z"
  PS-Simulink Converter2/1 -> Mux/2  "y"
  PS-Simulink Converter1/1 -> Mux/1  "x"
  Constant1/1 -> S-Function/3
  Integrator/1 -> S-Function/9
  scaling/1 -> S-Function/8
  road/1 -> S-Function/7
  add signal names/1(Out1) -> varinf/1  "varinf"
  S-Function/3 -> add signal names/1(In1)
  S-Function/4 -> Integrator/1
  PS-Simulink Converter/1 -> Reshape/1
  Mux1/1 -> S-Function/5
  Mux2/1 -> S-Function/4
  Constant2/1 -> S-Function/6
  PS-Simulink Converter10/1 -> Display/1
  PS-Simulink Converter11/1 -> Display1/1
  connections:
  Transform Sensor-WorldCS/LConn1 -- World Frame/RConn1 -- Transform Sensor-LocalBodyCS/LConn1
  Inertia/RConn1 -- Transform Spin Axis/LConn1 -- Transform Sensor-WorldCS/RConn1 -- Transform Sensor-LocalBodyCS/RConn1 -- External Force and Torque/RConn1 -- Transform Geometry/LConn1 -- Inertia Sensor1/LConn2
  Transform Geometry/RConn1 -- Rim/RConn1 -- Tire/RConn1
  Transform Sensor-LocalBodyCS/RConn7 -- PS-Simulink Converter9/LConn1
  Transform Sensor-LocalBodyCS/RConn6 -- PS-Simulink Converter8/LConn1
  Transform Sensor-LocalBodyCS/RConn5 -- PS-Simulink Converter7/LConn1
  Transform Sensor-LocalBodyCS/RConn4 -- PS-Simulink Converter6/LConn1
  Transform Sensor-LocalBodyCS/RConn3 -- PS-Simulink Converter5/LConn1
  Transform Sensor-LocalBodyCS/RConn2 -- PS-Simulink Converter4/LConn1
  Transform Sensor-WorldCS/RConn5 -- PS-Simulink Converter3/LConn1
  Transform Sensor-WorldCS/RConn4 -- PS-Simulink Converter2/LConn1
  Transform Sensor-WorldCS/RConn3 -- PS-Simulink Converter1/LConn1
  Transform Sensor-WorldCS/RConn2 -- PS-Simulink Converter/LConn1
  Simulink-PS Converter/RConn1 -- External Force and Torque/LConn1
  Simulink-PS Converter1/RConn1 -- External Force and Torque/LConn2
  Transform Spin Axis/RConn1 -- wheel/RConn1 -- Inertia Sensor1/LConn1
  PS-Simulink Converter10/LConn1 -- Inertia Sensor1/RConn2
  Inertia Sensor1/RConn1 -- PS-Simulink Converter11/LConn1

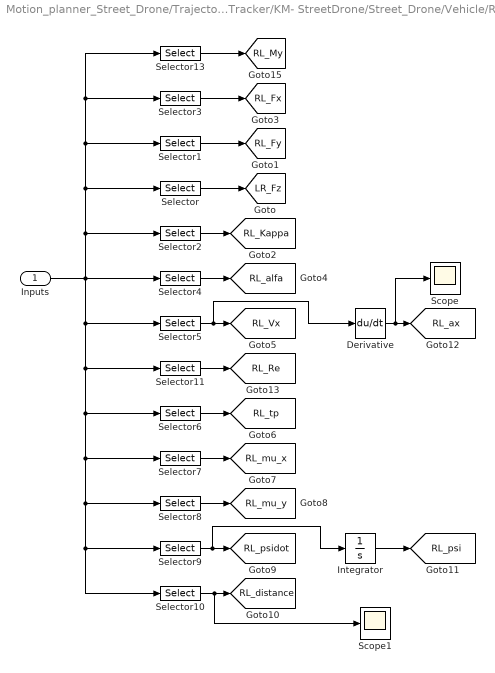
== system Motion_planner_Street_Drone/Trajectory Tracker/KM- StreetDrone/Street_Drone/Vehicle/RL_Wheel/For Validation ==
  Inputs : Inport
  Derivative : Derivative
  Integrator : Integrator
  Scope : Scope
  Scope1 : Scope
  Selector : Selector  InputPortWidth=40  IndexOptions=Index vector (dialog)  Indices=[3]  OutputSizes=1
  Selector1 : Selector  InputPortWidth=40  IndexOptions=Index vector (dialog)  Indices=[2]  OutputSizes=1
  Selector10 : Selector  InputPortWidth=40  IndexOptions=Index vector (dialog)  Indices=[28]  OutputSizes=1
  Selector11 : Selector  InputPortWidth=40  IndexOptions=Index vector (dialog)  Indices=[13]  OutputSizes=1
  Selector13 : Selector  InputPortWidth=40  IndexOptions=Index vector (dialog)  Indices=[5]  OutputSizes=1
  Selector2 : Selector  InputPortWidth=40  IndexOptions=Index vector (dialog)  Indices=[7]  OutputSizes=1
  Selector3 : Selector  InputPortWidth=40  IndexOptions=Index vector (dialog)  Indices=[1]  OutputSizes=1
  Selector4 : Selector  InputPortWidth=40  IndexOptions=Index vector (dialog)  Indices=[8]  OutputSizes=1
  Selector5 : Selector  InputPortWidth=40  IndexOptions=Index vector (dialog)  Indices=[11]  OutputSizes=1
  Selector6 : Selector  InputPortWidth=40  IndexOptions=Index vector (dialog)  Indices=[16]  OutputSizes=1
  Selector7 : Selector  InputPortWidth=40  IndexOptions=Index vector (dialog)  Indices=[17]  OutputSizes=1
  Selector8 : Selector  InputPortWidth=40  IndexOptions=Index vector (dialog)  Indices=[18]  OutputSizes=1
  Selector9 : Selector  InputPortWidth=40  IndexOptions=Index vector (dialog)  Indices=[24]  OutputSizes=1
  tag scope: LR_Fz=global, RL_Fx=global, RL_Fy=global, RL_Kappa=global, RL_My=global, RL_Re=global, RL_Vx=global, RL_alfa=global, RL_ax=global, RL_distance=global, RL_mu_x=global, RL_mu_y=global, RL_psi=global, RL_psidot=global, RL_tp=global
  wires:
  Selector13/1 -> [RL_My]
  Derivative/1 -> Scope/1, [RL_ax]
  Integrator/1 -> [RL_psi]
  Selector10/1 -> Scope1/1, [RL_distance]
  Selector9/1 -> [RL_psidot], Integrator/1
  Selector8/1 -> [RL_mu_y]
  Selector7/1 -> [RL_mu_x]
  Selector6/1 -> [RL_tp]
  Selector5/1 -> [RL_Vx], Derivative/1
  Selector4/1 -> [RL_alfa]
  Selector3/1 -> [RL_Fx]
  Selector2/1 -> [RL_Kappa]
  Selector1/1 -> [RL_Fy]
  Selector/1 -> [LR_Fz]
  Selector11/1 -> [RL_Re]
  Inputs/1 -> Selector11/1, Selector6/1, Selector7/1, Selector8/1, Selector9/1, Selector10/1, Selector5/1, Selector1/1, Selector3/1, Selector13/1, Selector/1, Selector2/1, Selector4/1

== system Motion_planner_Street_Drone/Trajectory Tracker/KM- StreetDrone/Street_Drone/Vehicle/RL_Wheel/Non-moving road ==
  omega2 : Constant  Value=zeros(18,1)
  road : Outport
  wires:
  omega2/1 -> road/1

== system Motion_planner_Street_Drone/Trajectory Tracker/KM- StreetDrone/Street_Drone/Vehicle/RL_Wheel/Scaling factors ==
  s_LKX : Constant  Value=LKX
  s_LKY : Constant  Value=LKY
  s_LKYC : Constant  Value=LKYC
  s_LKZC : Constant  Value=LKZC
  s_LMUX : Constant  Value=LMUX
  s_LMUY : Constant  Value=LMUY
  s_LTR : Constant  Value=LTR
  scaling_vector : Mux  Inputs=7
  scaling : Outport
  wires:
  scaling_vector/1 -> scaling/1
  s_LKZC/1 -> scaling_vector/7
  s_LTR/1 -> scaling_vector/6
  s_LKYC/1 -> scaling_vector/5
  s_LKY/1 -> scaling_vector/4
  s_LMUY/1 -> scaling_vector/3
  s_LKX/1 -> scaling_vector/2
  s_LMUX/1 -> scaling_vector/1

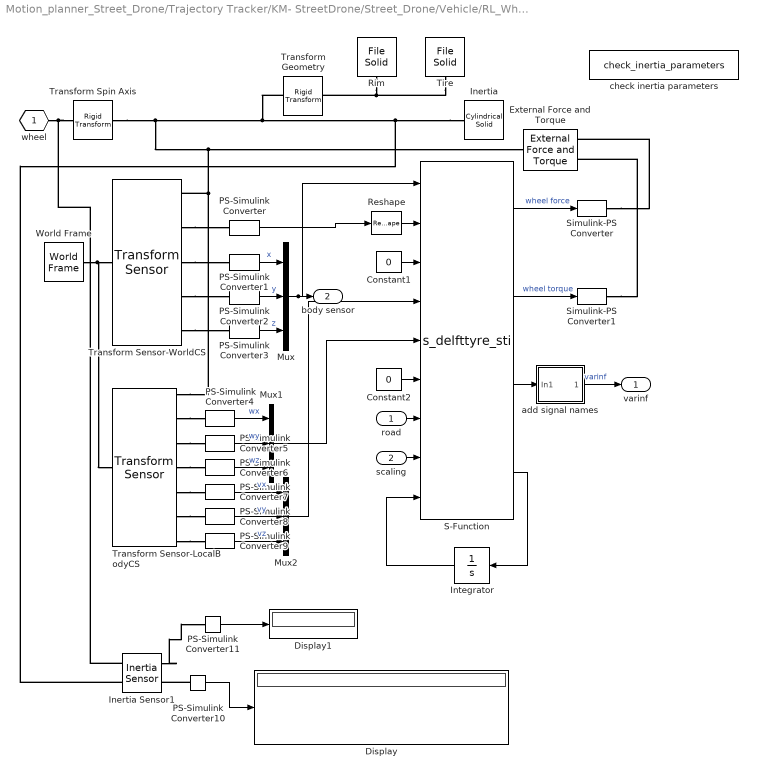
== system Motion_planner_Street_Drone/Trajectory Tracker/KM- StreetDrone/Street_Drone/Vehicle/RL_Wheel/SimMechanics2G Wheel + tyre ==
  road : Inport
  scaling : Inport  Port=2
  Constant1 : Constant  Value=0
  Constant2 : Constant  Value=0
  Display : Display
  Display1 : Display
  External Force and Torque : sm_lib/Forces and Torques/External Force and Torque  ForceResolutionFrame=AttachedFrame  EnableForceX=off  EnableForceY=off  EnableForceZ=off  EnableForce=on  TorqueResolutionFrame=AttachedFrame  EnableTorqueX=off  EnableTorqueY=off  EnableTorqueZ=off  EnableTorque=on
  Inertia : sm_lib/Body Elements/Cylindrical Solid  GraphicAmbientColor=[0.15 0.15 0.15 1.0]  BasedOnType=Density  CenterOfMass=[0 0 0]  CenterOfMassUnits=m  GraphicDiffuseColor=[0.2 0.8 1.0]  CylinderLength=0.001  CylinderLengthUnits=m  CylinderRadius=0.001  CylinderRadiusUnits=m  Density=1000  DensityUnits=kg/(m^3)  DoExposeReferenceFrame=on  GraphicEmissiveColor=[0.0 0.0 0.0 1.0]  ExportEntireGeometry=off  SerializedFrames=<Frames/>  MarkerShape=Sphere  MarkerSize=10  GraphicType=FromGeometry  InertiaType=Custom  Mass=mass  MassUnits=kg  MomentsOfInertia=[Imat(1,1) Imat(2,2) Imat(3,3)]  MomentsOfInertiaUnits=kg*m^2  GraphicOpacity=1.0  ProductsOfInertia=[0 0 0]  ProductsOfInertiaUnits=kg*m^2  GraphicShininess=75  GraphicSpecularColor=[0.5 0.5 0.5 1.0]  GraphicVisPropType=SimpleVisualProperties
  Inertia Sensor1 : sm_lib/Body Elements/Inertia Sensor  SensorExtent=BodyGroup  SpanWeldJoints=off  ExcludeGroundedBodies=off  MeasurementFrame=Custom  SenseMass=on  SenseCenterOfMass=off  SenseInertiaMatrix=on  SenseCenteredInertiaMatrix=off  SensePrincipalInertiaMatrix=off  SenseRotationMatrix=off  GraphicType=PrincipalInertiaFrame  PrincipalInertiaFrameSize=20  GraphicVisPropType=SimpleVisualProperties  GraphicDiffuseColor=[0.5 0.5 0.5]  GraphicSpecularColor=[0.5 0.5 0.5 1.0]  GraphicAmbientColor=[0.15 0.15 0.15 1.0]  GraphicEmissiveColor=[0.0 0.0 0.0 1.0]  GraphicShininess=75  GraphicOpacity=1.0
      settings: SourceProductBaseCode=MS
  Integrator : Integrator  InitialCondition=zeros(1,40)
  Mux : Mux  Inputs=3
  Mux1 : Mux  Inputs=3
  Mux2 : Mux  Inputs=3
  PS-Simulink Converter{,1..9} (10 alike) : nesl_utility/PS-Simulink Converter  PhysicalDomain=network_engine_domain  SubClassName=ps_output  LeftPortType=input  RightPortType=output  PseudoPeriodic=off  Frequencies=[]  Unit=1  AffineConversion=off
  PS-Simulink Converter10 : nesl_utility/PS-Simulink Converter  PhysicalDomain=network_engine_domain  SubClassName=ps_output  LeftPortType=input  RightPortType=output  PseudoPeriodic=off  Frequencies=[]  Unit=inherit  AffineConversion=off
  PS-Simulink Converter11 : nesl_utility/PS-Simulink Converter  PhysicalDomain=network_engine_domain  SubClassName=ps_output  LeftPortType=input  RightPortType=output  PseudoPeriodic=off  Frequencies=[]  Unit=inherit  AffineConversion=off
  Reshape : Reshape
  Rim : sm_lib/Body Elements/File Solid  ExtGeomFileName=D:\Project\PATH PLANNER STREET DRONE - 618341\CAD geometry\Rim_Back.stl  UnitType=Custom  ExtGeomFileUnits=mm  StepReaderType=HEX  ExportEntireGeometry=off  InertiaType=Custom  Mass=0  MassUnits=kg  CenterOfMass=[0 0 0]  CenterOfMassUnits=m  MomentsOfInertia=[0 0 0]  MomentsOfInertiaUnits=kg*m^2  ProductsOfInertia=[0 0 0]  ProductsOfInertiaUnits=kg*m^2  BasedOnType=Density  Density=1000  DensityUnits=kg/(m^3)  DoExposeReferenceFrame=on  SerializedFrames=<Frames/>  GraphicType=FromGeometry  MarkerShape=Sphere  MarkerSize=10  MarkerSizeUnits=m  GraphicVisPropType=SimpleVisualProperties  GraphicDiffuseColor=[0.8 0.8 0.8]  GraphicSpecularColor=[0.5 0.5 0.5 1.0]  GraphicAmbientColor=[0.15 0.15 0.15 1.0]  GraphicEmissiveColor=[0.0 0.0 0.0 1.0]  GraphicShininess=75  GraphicOpacity=1.0
  S-Function : S-Function  FunctionName=s_delfttyre_sti  Parameters=iswtch idtyre idroad tpfname_dummy rdfname typarr  SFunctionDeploymentMode=off  EnableBusSupport=off
  Simulink-PS Converter : nesl_utility/Simulink-PS Converter  PhysicalDomain=network_engine_domain  SubClassName=ps_input  LeftPortType=input  RightPortType=output  PseudoPeriodic=off  Frequencies=[]  NoiseDistribution=none  NoiseParameters=[]  Unit=1  AffineConversion=off  FilteringAndDerivatives=zero  SimscapeFilterOrder=1  InputFilterTimeConstant=0.001  UdotUserProvided=1
  Simulink-PS Converter1 : nesl_utility/Simulink-PS Converter  PhysicalDomain=network_engine_domain  SubClassName=ps_input  LeftPortType=input  RightPortType=output  PseudoPeriodic=off  Frequencies=[]  NoiseDistribution=none  NoiseParameters=[]  Unit=1  AffineConversion=off  FilteringAndDerivatives=zero  SimscapeFilterOrder=1  InputFilterTimeConstant=0.001  UdotUserProvided=1
  Tire : sm_lib/Body Elements/File Solid  ExtGeomFileName=D:\Project\PATH PLANNER STREET DRONE - 618341\CAD geometry\Tire_Back.stl  UnitType=Custom  ExtGeomFileUnits=mm  StepReaderType=HEX  ExportEntireGeometry=off  InertiaType=Custom  Mass=0  MassUnits=kg  CenterOfMass=[0 0 0]  CenterOfMassUnits=m  MomentsOfInertia=[0 0 0]  MomentsOfInertiaUnits=kg*m^2  ProductsOfInertia=[0 0 0]  ProductsOfInertiaUnits=kg*m^2  BasedOnType=Density  Density=1000  DensityUnits=kg/(m^3)  DoExposeReferenceFrame=on  SerializedFrames=<Frames/>  GraphicType=FromGeometry  MarkerShape=Sphere  MarkerSize=10  MarkerSizeUnits=m  GraphicVisPropType=SimpleVisualProperties  GraphicDiffuseColor=[0.5 0.5 0.5]  GraphicSpecularColor=[0.5 0.5 0.5 1.0]  GraphicAmbientColor=[0.15 0.15 0.15 1.0]  GraphicEmissiveColor=[0.0 0.0 0.0 1.0]  GraphicShininess=75  GraphicOpacity=1.0
  Transform Geometry : sm_lib/Frames and Transforms/Rigid Transform  TranslationMethod=StandardAxis  TranslationStandardOffset=(1-2*fliplr)*0.125  TranslationLengthUnit=m  TranslationStandardAxis=+Y  TranslationCartesianOffset=[0 0 0]  TranslationROffset=0  TranslationROffsetUnits=m  TranslationZOffset=0  TranslationZOffsetUnits=m  TranslationThetaOffset=0  TranslationThetaOffsetUnits=deg  RotationMethod=StandardAxis  RotationAngleUnits=deg  RotationStandardAxis=+X  RotationAngle=fliplr*180-90  RotationArbitraryAxis=[0 0 1]  FollAlignAxisA=+X  BaseAlignAxisA=+Y  FollAlignAxisB=+Y  BaseAlignAxisB=+Z  RotationSequenceAxes=FollowerAxes  RotationSequence=XYX  RotationSequenceAngles=[0 0 0]  RotationSequenceAnglesUnits=deg  RotationMatrix=[1 0 0; 0 1 0; 0 0 1]
  Transform Sensor-LocalBodyCS : sm_lib/Frames and Transforms/Transform Sensor  MeasurementFrame=NonRotatingFollower  SenseAngle=off  SenseAxis=off  SenseAngle1=off  SenseAngle2=off  SenseAngle3=off  SenseQ=off  SenseR=off  SenseOmegaX=on  SenseOmegaY=on  SenseOmegaZ=on  SenseOmega1=off  SenseOmega2=off  SenseOmega3=off  SenseQDot=off  SenseRDot=off  SenseAlphaX=off  SenseAlphaY=off  SenseAlphaZ=off  SenseAlpha1=off  SenseAlpha2=off  SenseAlpha3=off  SenseQDDot=off  SenseRDDot=off  SenseX=off  SenseY=off  SenseZ=off  SenseRad=off  SenseAzim=off  SenseDist=off  SenseInc=off  SenseXDot=on  SenseYDot=on  SenseZDot=on  SenseRadDot=off  SenseAzimDot=off  SenseDistDot=off  SenseIncDot=off  SenseXDDot=off  SenseYDDot=off  SenseZDDot=off  SenseRadDDot=off  SenseAzimDDot=off  SenseDistDDot=off  SenseIncDDot=off
  Transform Sensor-WorldCS : sm_lib/Frames and Transforms/Transform Sensor  MeasurementFrame=World  SenseAngle=off  SenseAxis=off  SenseAngle1=off  SenseAngle2=off  SenseAngle3=off  SenseQ=off  SenseR=on  SenseOmegaX=off  SenseOmegaY=off  SenseOmegaZ=off  SenseOmega1=off  SenseOmega2=off  SenseOmega3=off  SenseQDot=off  SenseRDot=off  SenseAlphaX=off  SenseAlphaY=off  SenseAlphaZ=off  SenseAlpha1=off  SenseAlpha2=off  SenseAlpha3=off  SenseQDDot=off  SenseRDDot=off  SenseX=on  SenseY=on  SenseZ=on  SenseRad=off  SenseAzim=off  SenseDist=off  SenseInc=off  SenseXDot=off  SenseYDot=off  SenseZDot=off  SenseRadDot=off  SenseAzimDot=off  SenseDistDot=off  SenseIncDot=off  SenseXDDot=off  SenseYDDot=off  SenseZDDot=off  SenseRadDDot=off  SenseAzimDDot=off  SenseDistDDot=off  SenseIncDDot=off
  Transform Spin Axis : sm_lib/Frames and Transforms/Rigid Transform  TranslationMethod=None  TranslationStandardOffset=0  TranslationLengthUnit=m  TranslationStandardAxis=+Z  TranslationCartesianOffset=[0 0 0]  TranslationROffset=0  TranslationROffsetUnits=m  TranslationZOffset=0  TranslationZOffsetUnits=m  TranslationThetaOffset=0  TranslationThetaOffsetUnits=deg  RotationMethod=StandardAxis  RotationAngleUnits=deg  RotationStandardAxis=-X  RotationAngle=90  RotationArbitraryAxis=[0 0 1]  FollAlignAxisA=+X  BaseAlignAxisA=+Y  FollAlignAxisB=+Y  BaseAlignAxisB=+Z  RotationSequenceAxes=FollowerAxes  RotationSequence=XYX  RotationSequenceAngles=[0 0 0]  RotationSequenceAnglesUnits=deg  RotationMatrix=[1 0 0; 0 1 0; 0 0 1]
  World Frame : sm_lib/Frames and Transforms/World Frame
  add signal names : Subsystem
  check inertia parameters : M-S-Function  Priority=1  FunctionName=check_inertia_parameters  Parameters=tpfname1, rdfname1, typarr1  mask{tpfname1=tpfname_dummy, rdfname1=rdfname, typarr1=typarr}
      mask prompts: tpfname1 "Tyre Property File"; rdfname1 "Road Data File"; typarr1 "typarr"
      mask help: Checks Inertia parameters as calculated in mask
  wheel : PMIOPort  Side=Left
  varinf : Outport
  body sensor : Outport  Port=2
  wires:
  Reshape/1 -> S-Function/2
  S-Function/1 -> Simulink-PS Converter/1  "wheel force"
  S-Function/2 -> Simulink-PS Converter1/1  "wheel torque"
  Mux/1 -> S-Function/1, body sensor/1
  PS-Simulink Converter9/1 -> Mux2/3  "vz"
  PS-Simulink Converter8/1 -> Mux2/2  "vy"
  PS-Simulink Converter7/1 -> Mux2/1  "vx"
  PS-Simulink Converter6/1 -> Mux1/3  "wz"
  PS-Simulink Converter5/1 -> Mux1/2  "wy"
  PS-Simulink Converter4/1 -> Mux1/1  "wx"
  PS-Simulink Converter3/1 -> Mux/3  "z"
  PS-Simulink Converter2/1 -> Mux/2  "y"
  PS-Simulink Converter1/1 -> Mux/1  "x"
  Constant1/1 -> S-Function/3
  Integrator/1 -> S-Function/9
  scaling/1 -> S-Function/8
  road/1 -> S-Function/7
  add signal names/1(Out1) -> varinf/1  "varinf"
  S-Function/3 -> add signal names/1(In1)
  S-Function/4 -> Integrator/1
  PS-Simulink Converter/1 -> Reshape/1
  Mux1/1 -> S-Function/5
  Mux2/1 -> S-Function/4
  Constant2/1 -> S-Function/6
  PS-Simulink Converter10/1 -> Display/1
  PS-Simulink Converter11/1 -> Display1/1
  connections:
  Transform Sensor-WorldCS/LConn1 -- World Frame/RConn1 -- Transform Sensor-LocalBodyCS/LConn1
  Inertia/RConn1 -- Transform Spin Axis/LConn1 -- Transform Sensor-WorldCS/RConn1 -- Transform Sensor-LocalBodyCS/RConn1 -- External Force and Torque/RConn1 -- Transform Geometry/LConn1 -- Inertia Sensor1/LConn2
  Transform Geometry/RConn1 -- Rim/RConn1 -- Tire/RConn1
  Transform Sensor-LocalBodyCS/RConn7 -- PS-Simulink Converter9/LConn1
  Transform Sensor-LocalBodyCS/RConn6 -- PS-Simulink Converter8/LConn1
  Transform Sensor-LocalBodyCS/RConn5 -- PS-Simulink Converter7/LConn1
  Transform Sensor-LocalBodyCS/RConn4 -- PS-Simulink Converter6/LConn1
  Transform Sensor-LocalBodyCS/RConn3 -- PS-Simulink Converter5/LConn1
  Transform Sensor-LocalBodyCS/RConn2 -- PS-Simulink Converter4/LConn1
  Transform Sensor-WorldCS/RConn5 -- PS-Simulink Converter3/LConn1
  Transform Sensor-WorldCS/RConn4 -- PS-Simulink Converter2/LConn1
  Transform Sensor-WorldCS/RConn3 -- PS-Simulink Converter1/LConn1
  Transform Sensor-WorldCS/RConn2 -- PS-Simulink Converter/LConn1
  Simulink-PS Converter/RConn1 -- External Force and Torque/LConn1
  Simulink-PS Converter1/RConn1 -- External Force and Torque/LConn2
  Transform Spin Axis/RConn1 -- wheel/RConn1 -- Inertia Sensor1/LConn1
  PS-Simulink Converter10/LConn1 -- Inertia Sensor1/RConn2
  Inertia Sensor1/RConn1 -- PS-Simulink Converter11/LConn1
